simulink model "Practica_control_ej_1_2_5"  (R2024b)
settings: Solver=VariableStepAuto  StartTime=0.0  StopTime=3  RelTol=1e-3
model workspace (MAT data in the model file):
  A = 10
  B1 = 0.04
  B2 = 2
  J = 0.025
  Kp = 1
  Kt = 0.86
  Kw = 0.17
  La = 0.04
  Ra = 2.4
  k = Simulink.Parameter
  k.Value = 500
  k.Complexity = 'real'
  k.Dimensions = [1 1]
  k.DataType = 'auto'
  r = 0.1
values from neighbouring files (symbols this model uses):
  k = 0.2    [practica_control_1_2.m]    (also in practica_control_1_2_ej2.m)
settings Model: Creator=Carlos  LastModifiedBy=carlos

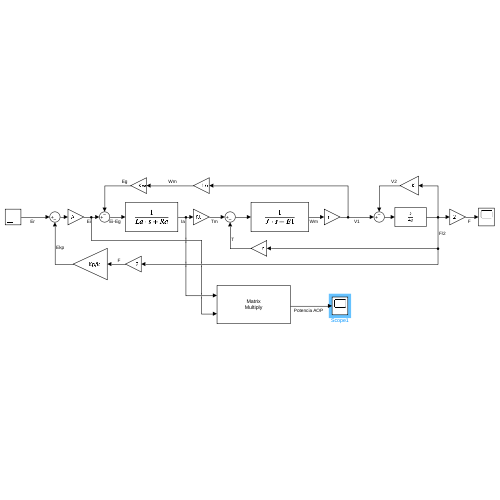
[thumbnail: Simulink's stored preview of the top-level diagram]
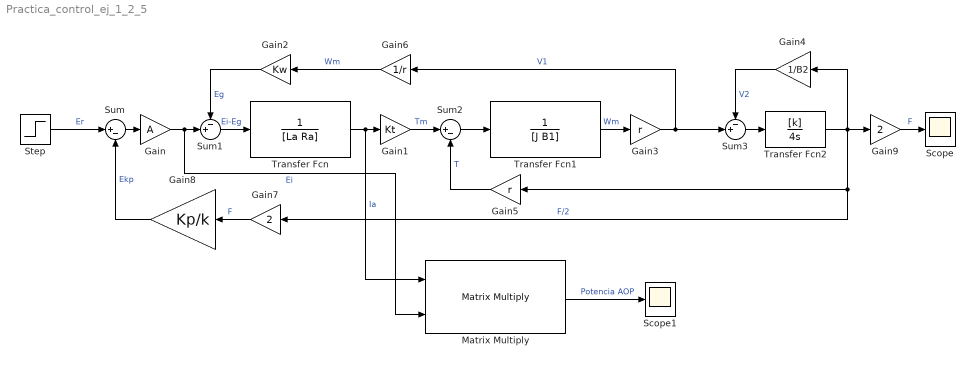
== system Practica_control_ej_1_2_5 ==
  Gain : Gain  Gain=A
  Gain1 : Gain  Gain=Kt
  Gain2 : Gain  Gain=Kw
  Gain3 : Gain  Gain=r
  Gain4 : Gain  Gain=1/B2
  Gain5 : Gain  Gain=r
  Gain6 : Gain  Gain=1/r
  Gain7 : Gain  Gain=2
  Gain8 : Gain  Gain=Kp/k
  Gain9 : Gain  Gain=2
  Matrix Multiply : Product  Multiplication=Matrix(*)
  Scope : Scope
  Scope1 : Scope
  Step : Step  SampleTime=0
  Sum : Sum  Inputs=|+-
  Sum1 : Sum  Inputs=-+|
  Sum2 : Sum  Inputs=|+-
  Sum3 : Sum  Inputs=-+|
  Transfer Fcn : TransferFcn  Denominator=[La Ra]
  Transfer Fcn1 : TransferFcn  Denominator=[J B1]
  Transfer Fcn2 : TransferFcn  Numerator=[k]  Denominator=[4 0]
  wires:
  Step/1 -> Sum/1  "Er"
  Sum/1 -> Gain/1
  Gain8/1 -> Sum/2  "Ekp"
  Sum1/1 -> Transfer Fcn/1  "Ei-Eg"
  Transfer Fcn/1 -> Matrix Multiply/1, Gain1/1  "Ia"
  Gain1/1 -> Sum2/1  "Tm"
  Gain6/1 -> Gain2/1  "Wm"
  Gain5/1 -> Sum2/2  "T"
  Sum2/1 -> Transfer Fcn1/1
  Transfer Fcn1/1 -> Gain3/1  "Wm"
  Gain3/1 -> Gain6/1, Sum3/2  "V1"
  Sum3/1 -> Transfer Fcn2/1
  Transfer Fcn2/1 -> Gain7/1, Gain5/1, Gain4/1, Gain9/1  "F/2"
  Gain7/1 -> Gain8/1  "F"
  Gain9/1 -> Scope/1  "F"
  Gain4/1 -> Sum3/1  "V2"
  Gain2/1 -> Sum1/1  "Eg"
  Gain/1 -> Matrix Multiply/2, Sum1/2  "Ei"
  Matrix Multiply/1 -> Scope1/1  "Potencia AOP"
